simulink model "Q2_Part_b3"  (R2016b)
settings: Solver=VariableStepAuto  StartTime=0.0  StopTime=5  RelTol=1e-8  AbsTol=1e-8
values from neighbouring files (symbols this model uses):
  P1 = P    [CSD_Assignment_2_Script.m]
  P2 = tf(1,[1 0])    [CSD_Assignment_2_Script.m]
libraries: cstblocks x2
settings Model: Creator=nadav  LastModifiedBy=nadav

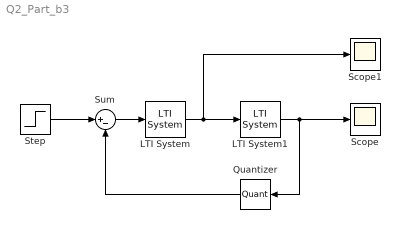
== system Q2_Part_b3 ==
  LTI System : cstblocks/LTI System  sys=C  IC=[]
  LTI System1 : cstblocks/LTI System  sys=P1*P2  IC=[]
  Quantizer : Quantizer  QuantizationInterval=enc_res  LinearizeAsGain=off
  Scope : Scope
  Scope1 : Scope
  Step : Step  Time=0  SampleTime=0
  Sum : Sum  Inputs=|+-
  wires:
  LTI System/1 -> Scope1/1, LTI System1/1
  Sum/1 -> LTI System/1
  LTI System1/1 -> Quantizer/1, Scope/1
  Step/1 -> Sum/1
  Quantizer/1 -> Sum/2
